simulink model "Quadcopter_nonlinear_Roll_Pitch"  (R2020a)
settings: Solver=ode4  StartTime=0.0  StopTime=10.0  FixedStep=0.02  RelTol=1e-3
InitFcn:
  | load_data;
values from neighbouring files (symbols this model uses):
  A1 = (h_cg * g * m_tot) / (m_tot * h_cg^2 + J_xx)    [QuadConstants.m]    (also in roll_parameter_estimation_result.m = 4.62576573735; roll_pitch_parameter_estimation.m = 6.52172868745)
  A3 = (b * d_cg) / (m_tot * h_cg^2 + J_xx)    [QuadConstants.m]    (also in roll_parameter_estimation_result.m = 5.47149559873e-05; roll_pitch_parameter_estimation.m = 5.18692283683e-05)
  A4 = (J_R) / (m_tot * h_cg^2 + J_xx)    [QuadConstants.m]    (also in roll_pitch_parameter_estimation.m = 0.00249993776858)
  A5 = (m1 * g * miu_k * r_x) / (m_tot * h_cg^2 + J_xx)    [QuadConstants.m]    (also in roll_parameter_estimation_result.m = 0.0125335544194; roll_pitch_parameter_estimation.m = -0.25964581952)
  A6 = 0.628891443554123    (= 0.628891443554)    [roll_parameter_estimation_result.m]    (also in roll_pitch_parameter_estimation.m = 1.37409031322)
  b = 3.12e-5    (= 3.12e-05)    [QuadParameter.m]    (also in QuadParameter_v1.m = 3.13e-05)
  B6 = 3.49728    [pitch_parameter_estiation_result.m]    (also in pitch_parameter_estiation_result_II.m = 4.42876359313; roll_pitch_parameter_estimation.m = 4.42876359313)
  d_cg = 0.295    [QuadParameter.m]    (also in QuadParameter_v1.m = 0.2)
  g = 9.81    [QuadParameter.m]
  h_cg = 0.0078    [QuadParameter.m]
  init_I = data_I(1, :)    [PS_I.m]
  init_II = data_II(1, :)    [PS_II.m]
  init_III = data_III(1, :)    [PS_III.m]
  init_IV = data_IV(1, :)    [PS_IV.m]
  init_IX = data_IX(1, :)    [PS_IX.m]
  init_V = data_V(1, :)    [PS_V.m]
  init_VI = data_VI(1, :)    [PS_VI.m]
  init_VII = data_VII(1, :)    [PS_VII.m]
  init_X = data_X(1, :)    [PS_X.m]
  J_R = 4.439e-5    (= 4.439e-05)    [QuadParameter.m]
  J_yy = 0.03066    [QuadParameter.m]
  m2 = 1.074    [QuadParameter.m]
  m_tot = 1.774    [QuadParameter.m]
  miu_k = 0.002    [QuadParameter.m]
  Omega_I = Omega(1, :)    [PS_I.m]
  Omega_II = Omega(1, :)    [PS_II.m]
  Omega_III = Omega(1, :)    [PS_III.m]
  Omega_IV = Omega(1, :)    [PS_IV.m]
  Omega_IX = Omega(1, :)    [PS_IX.m]
  Omega_V = Omega(1, :)    [PS_V.m]
  Omega_VI = Omega(1, :)    [PS_VI.m]
  Omega_VII = Omega(1, :)    [PS_VII.m]
  Omega_X = Omega(1, :)    [PS_X.m]
  r_y = 0.01    [QuadParameter.m]
undefined symbols (not defined in the file or in its folder): magnitude
(part 2 of 3)

== system Quadcopter_nonlinear_Roll_Pitch/Quadcopter 2DOF (Roll-Pitch) Nonlinear System1/Quad System/dot(x1)/1 ==
  X : Inport
  Demux : Demux  Outputs=3
  Selector : Selector  InputPortWidth=4  IndexOptions=Index vector (dialog)  Indices=[1 2 4]  OutputSizes=1
  Subsystem : Subsystem
  x5sin(x1)tan(x2) : Outport
  wires:
  Demux/2 -> Subsystem/2(x2)  "x2"
  X/1 -> Selector/1  "x"
  Demux/1 -> Subsystem/1(x1)  "x1"
  Demux/3 -> Subsystem/3(x5)  "x5"
  Subsystem/1(x5sin(x1)tan(x2)) -> x5sin(x1)tan(x2)/1
  Selector/1 -> Demux/1

== system Quadcopter_nonlinear_Roll_Pitch/Quadcopter 2DOF (Roll-Pitch) Nonlinear System1/Quad System/dot(x1)/Subsystem1 ==
  X : Inport
  Selector : Selector  InputPortWidth=4  IndexOptions=Index vector (dialog)  Indices=[3]  OutputSizes=1
  x4 : Outport
  wires:
  Selector/1 -> x4/1
  X/1 -> Selector/1

== system Quadcopter_nonlinear_Roll_Pitch/Quadcopter 2DOF (Roll-Pitch) Nonlinear System1/Quad System/dot(x2)/1 ==
  X : Inport
  Demux : Demux  Outputs=2
  Selector : Selector  InputPortWidth=4  IndexOptions=Index vector (dialog)  Indices=[1 4]  OutputSizes=1
  Subsystem : Subsystem
  x5cos(x1) : Outport
  wires:
  X/1 -> Selector/1  "x"
  Demux/1 -> Subsystem/1(x1)  "x1"
  Demux/2 -> Subsystem/2(x5)  "x5"
  Subsystem/1(Out1) -> x5cos(x1)/1
  Selector/1 -> Demux/1

== system Quadcopter_nonlinear_Roll_Pitch/Quadcopter 2DOF (Roll-Pitch) Nonlinear System1/Quad System/dot(x4)/1 ==
  X : Inport
  Demux : Demux  Outputs=2
  Selector : Selector  InputPortWidth=4  IndexOptions=Index vector (dialog)  Indices=[1 2]  OutputSizes=1
  Subsystem : Subsystem
  A1cos(x2)sin(x1) : Outport
  wires:
  Demux/1 -> Subsystem/1(x1)  "x1"
  Subsystem/1(A1cos(x2)sin(x1)) -> A1cos(x2)sin(x1)/1
  Demux/2 -> Subsystem/2(x2)  "x2"
  X/1 -> Selector/1  "x"
  Selector/1 -> Demux/1

== system Quadcopter_nonlinear_Roll_Pitch/Quadcopter 2DOF (Roll-Pitch) Nonlinear System1/Quad System/dot(x4)/2 ==
  X : Inport
  Selector : Selector  InputPortWidth=4  IndexOptions=Index vector (dialog)  Indices=[1]  OutputSizes=1
  Subsystem : Subsystem
  Moment a : Outport
  wires:
  Selector/1 -> Subsystem/1(x1)  "x1"
  Subsystem/1(Moment_a) -> Moment a/1
  X/1 -> Selector/1  "x"

== system Quadcopter_nonlinear_Roll_Pitch/Quadcopter 2DOF (Roll-Pitch) Nonlinear System1/Quad System/dot(x4)/3 ==
  X : Inport
  Selector : Selector  InputPortWidth=4  IndexOptions=Index vector (dialog)  Indices=[3]  OutputSizes=1
  Subsystem : Subsystem
  "-A5x4/|x4| " : Outport
  wires:
  Subsystem/1("-A5x4/|x4| ") -> "-A5x4/|x4| "/1
  Selector/1 -> Subsystem/1(x4)
  X/1 -> Selector/1  "x"

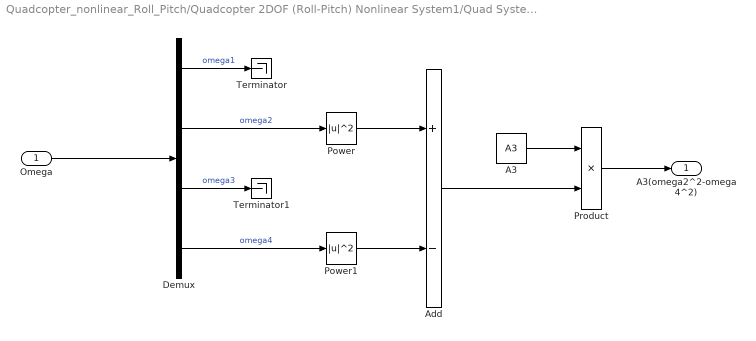
== system Quadcopter_nonlinear_Roll_Pitch/Quadcopter 2DOF (Roll-Pitch) Nonlinear System1/Quad System/dot(x4)/Subsystem ==
  Omega : Inport
  A3 : Constant  Value=A3
  Add : Sum  Inputs=+-
  Demux : Demux
  Power : Math  Operator=magnitude^2  SaturateOnIntegerOverflow=on
  Power1 : Math  Operator=magnitude^2  SaturateOnIntegerOverflow=on
  Product : Product
  Terminator : Terminator
  Terminator1 : Terminator
  A3(omega2^2-omega4^2) : Outport
  wires:
  Product/1 -> A3(omega2^2-omega4^2)/1
  Power1/1 -> Add/2
  Demux/2 -> Power/1  "omega2"
  Demux/4 -> Power1/1  "omega4"
  Add/1 -> Product/2
  Power/1 -> Add/1
  A3/1 -> Product/1
  Omega/1 -> Demux/1
  Demux/3 -> Terminator1/1  "omega3"
  Demux/1 -> Terminator/1  "omega1"

== system Quadcopter_nonlinear_Roll_Pitch/Quadcopter 2DOF (Roll-Pitch) Nonlinear System1/Quad System/dot(x4)/Subsystem1 ==
  X : Inport
  Omega : Inport  Port=2
  A4 : Constant  Value=A4
  Add : Sum  Inputs=+-+-
  Demux : Demux
  Product : Product  Inputs=3
  Selector : Selector  InputPortWidth=4  IndexOptions=Index vector (dialog)  Indices=[4]  OutputSizes=1
  A4x5(omega1-omega2+omega3-omega4) : Outport
  wires:
  Omega/1 -> Demux/1
  Demux/1 -> Add/1  "omega1"
  Demux/2 -> Add/2  "omega2"
  Demux/3 -> Add/3  "omega3"
  Demux/4 -> Add/4  "omega4"
  Add/1 -> Product/1
  A4/1 -> Product/2
  Product/1 -> A4x5(omega1-omega2+omega3-omega4)/1
  Selector/1 -> Product/3
  X/1 -> Selector/1  "x"

== system Quadcopter_nonlinear_Roll_Pitch/Quadcopter 2DOF (Roll-Pitch) Nonlinear System1/Quad System/dot(x5)/1 ==
  X : Inport
  Selector : Selector  InputPortWidth=4  IndexOptions=Index vector (dialog)  Indices=[2]  OutputSizes=1
  Subsystem : Subsystem
  B1sin(x2) : Outport
  wires:
  Subsystem/1(B1sin(x2)) -> B1sin(x2)/1
  Selector/1 -> Subsystem/1(x2)
  X/1 -> Selector/1  "x"

== system Quadcopter_nonlinear_Roll_Pitch/Quadcopter 2DOF (Roll-Pitch) Nonlinear System1/Quad System/dot(x5)/2 ==
  X : Inport
  Selector : Selector  InputPortWidth=4  IndexOptions=Index vector (dialog)  Indices=[2]  OutputSizes=1
  Subsystem : Subsystem
  Moment_a : Outport
  wires:
  X/1 -> Selector/1  "x"
  Subsystem/1(moment_a) -> Moment_a/1
  Selector/1 -> Subsystem/1(In1)

== system Quadcopter_nonlinear_Roll_Pitch/Quadcopter 2DOF (Roll-Pitch) Nonlinear System1/Quad System/dot(x5)/3 ==
  X : Inport
  Selector : Selector  InputPortWidth=4  IndexOptions=Index vector (dialog)  Indices=[4]  OutputSizes=1
  Subsystem : Subsystem
  "-B5x5/|x5| " : Outport
  wires:
  Selector/1 -> Subsystem/1(x5)  "x5"
  Subsystem/1("-B5x5/|x5| ") -> "-B5x5/|x5| "/1
  X/1 -> Selector/1  "x"

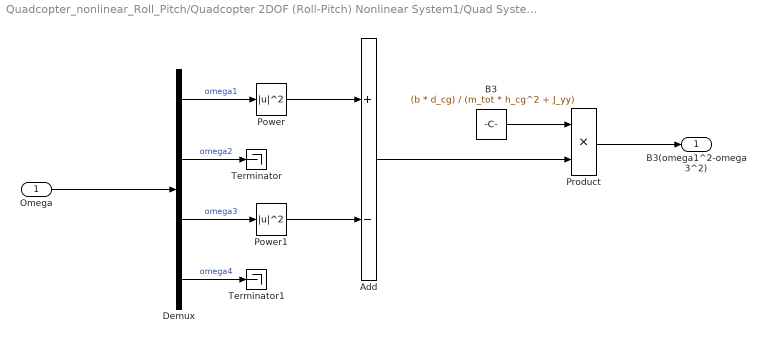
== system Quadcopter_nonlinear_Roll_Pitch/Quadcopter 2DOF (Roll-Pitch) Nonlinear System1/Quad System/dot(x5)/Subsystem ==
  Omega : Inport
  Add : Sum  Inputs=+-
  B3 : Constant  Value=(b * d_cg) / (m_tot * h_cg^2 + J_yy)
  Demux : Demux
  Power : Math  Operator=magnitude^2  SaturateOnIntegerOverflow=on
  Power1 : Math  Operator=magnitude^2  SaturateOnIntegerOverflow=on
  Product : Product
  Terminator : Terminator
  Terminator1 : Terminator
  B3(omega1^2-omega3^2) : Outport
  wires:
  Product/1 -> B3(omega1^2-omega3^2)/1
  Power1/1 -> Add/2
  Add/1 -> Product/2
  Power/1 -> Add/1
  B3/1 -> Product/1
  Omega/1 -> Demux/1
  Demux/3 -> Power1/1  "omega3"
  Demux/1 -> Power/1  "omega1"
  Demux/2 -> Terminator/1  "omega2"
  Demux/4 -> Terminator1/1  "omega4"

== system Quadcopter_nonlinear_Roll_Pitch/Quadcopter 2DOF (Roll-Pitch) Nonlinear System1/Quad System/dot(x5)/Subsystem1 ==
  X : Inport
  Omega : Inport  Port=2
  Add : Sum  Inputs=+-+-
  B4 : Constant  Value=(-J_R) / (m_tot * h_cg^2 + J_yy)
  Demux : Demux
  Product : Product  Inputs=3
  Selector : Selector  InputPortWidth=4  IndexOptions=Index vector (dialog)  Indices=[3]  OutputSizes=1
  B4x4(omega1-omega2+omega3-omega4) : Outport
  wires:
  Omega/1 -> Demux/1
  Demux/1 -> Add/1  "omega1"
  Demux/2 -> Add/2  "omega2"
  Demux/3 -> Add/3  "omega3"
  Demux/4 -> Add/4  "omega4"
  Add/1 -> Product/1
  B4/1 -> Product/2
  Product/1 -> B4x4(omega1-omega2+omega3-omega4)/1
  Selector/1 -> Product/3
  X/1 -> Selector/1  "x"

== system Quadcopter_nonlinear_Roll_Pitch/Quadcopter 2DOF (Roll-Pitch) Nonlinear System2/Quad System/dot(x1)/1 ==
  X : Inport
  Demux : Demux  Outputs=3
  Selector : Selector  InputPortWidth=4  IndexOptions=Index vector (dialog)  Indices=[1 2 4]  OutputSizes=1
  Subsystem : Subsystem
  x5sin(x1)tan(x2) : Outport
  wires:
  Demux/2 -> Subsystem/2(x2)  "x2"
  X/1 -> Selector/1  "x"
  Demux/1 -> Subsystem/1(x1)  "x1"
  Demux/3 -> Subsystem/3(x5)  "x5"
  Subsystem/1(x5sin(x1)tan(x2)) -> x5sin(x1)tan(x2)/1
  Selector/1 -> Demux/1

== system Quadcopter_nonlinear_Roll_Pitch/Quadcopter 2DOF (Roll-Pitch) Nonlinear System2/Quad System/dot(x1)/Subsystem1 ==
  X : Inport
  Selector : Selector  InputPortWidth=4  IndexOptions=Index vector (dialog)  Indices=[3]  OutputSizes=1
  x4 : Outport
  wires:
  Selector/1 -> x4/1
  X/1 -> Selector/1

== system Quadcopter_nonlinear_Roll_Pitch/Quadcopter 2DOF (Roll-Pitch) Nonlinear System2/Quad System/dot(x2)/1 ==
  X : Inport
  Demux : Demux  Outputs=2
  Selector : Selector  InputPortWidth=4  IndexOptions=Index vector (dialog)  Indices=[1 4]  OutputSizes=1
  Subsystem : Subsystem
  x5cos(x1) : Outport
  wires:
  X/1 -> Selector/1  "x"
  Demux/1 -> Subsystem/1(x1)  "x1"
  Demux/2 -> Subsystem/2(x5)  "x5"
  Subsystem/1(Out1) -> x5cos(x1)/1
  Selector/1 -> Demux/1

== system Quadcopter_nonlinear_Roll_Pitch/Quadcopter 2DOF (Roll-Pitch) Nonlinear System2/Quad System/dot(x4)/1 ==
  X : Inport
  Demux : Demux  Outputs=2
  Selector : Selector  InputPortWidth=4  IndexOptions=Index vector (dialog)  Indices=[1 2]  OutputSizes=1
  Subsystem : Subsystem
  A1cos(x2)sin(x1) : Outport
  wires:
  Demux/1 -> Subsystem/1(x1)  "x1"
  Subsystem/1(A1cos(x2)sin(x1)) -> A1cos(x2)sin(x1)/1
  Demux/2 -> Subsystem/2(x2)  "x2"
  X/1 -> Selector/1  "x"
  Selector/1 -> Demux/1

== system Quadcopter_nonlinear_Roll_Pitch/Quadcopter 2DOF (Roll-Pitch) Nonlinear System2/Quad System/dot(x4)/2 ==
  X : Inport
  Selector : Selector  InputPortWidth=4  IndexOptions=Index vector (dialog)  Indices=[1]  OutputSizes=1
  Subsystem : Subsystem
  Moment a : Outport
  wires:
  Selector/1 -> Subsystem/1(x1)  "x1"
  Subsystem/1(Moment_a) -> Moment a/1
  X/1 -> Selector/1  "x"

== system Quadcopter_nonlinear_Roll_Pitch/Quadcopter 2DOF (Roll-Pitch) Nonlinear System2/Quad System/dot(x4)/3 ==
  X : Inport
  Selector : Selector  InputPortWidth=4  IndexOptions=Index vector (dialog)  Indices=[3]  OutputSizes=1
  Subsystem : Subsystem
  "-A5x4/|x4| " : Outport
  wires:
  Subsystem/1("-A5x4/|x4| ") -> "-A5x4/|x4| "/1
  Selector/1 -> Subsystem/1(x4)
  X/1 -> Selector/1  "x"

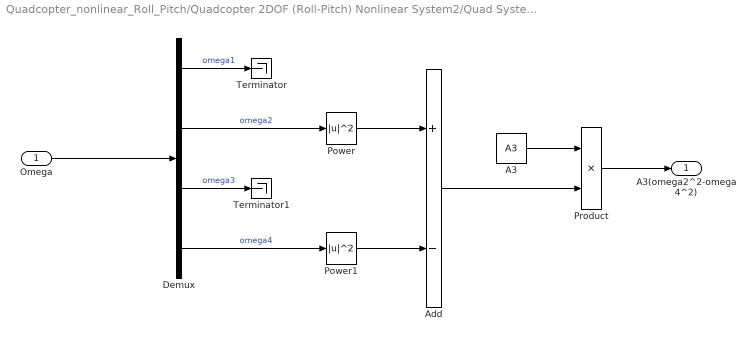
== system Quadcopter_nonlinear_Roll_Pitch/Quadcopter 2DOF (Roll-Pitch) Nonlinear System2/Quad System/dot(x4)/Subsystem ==
  Omega : Inport
  A3 : Constant  Value=A3
  Add : Sum  Inputs=+-
  Demux : Demux
  Power : Math  Operator=magnitude^2  SaturateOnIntegerOverflow=on
  Power1 : Math  Operator=magnitude^2  SaturateOnIntegerOverflow=on
  Product : Product
  Terminator : Terminator
  Terminator1 : Terminator
  A3(omega2^2-omega4^2) : Outport
  wires:
  Product/1 -> A3(omega2^2-omega4^2)/1
  Power1/1 -> Add/2
  Demux/2 -> Power/1  "omega2"
  Demux/4 -> Power1/1  "omega4"
  Add/1 -> Product/2
  Power/1 -> Add/1
  A3/1 -> Product/1
  Omega/1 -> Demux/1
  Demux/3 -> Terminator1/1  "omega3"
  Demux/1 -> Terminator/1  "omega1"

== system Quadcopter_nonlinear_Roll_Pitch/Quadcopter 2DOF (Roll-Pitch) Nonlinear System2/Quad System/dot(x4)/Subsystem1 ==
  X : Inport
  Omega : Inport  Port=2
  A4 : Constant  Value=A4
  Add : Sum  Inputs=+-+-
  Demux : Demux
  Product : Product  Inputs=3
  Selector : Selector  InputPortWidth=4  IndexOptions=Index vector (dialog)  Indices=[4]  OutputSizes=1
  A4x5(omega1-omega2+omega3-omega4) : Outport
  wires:
  Omega/1 -> Demux/1
  Demux/1 -> Add/1  "omega1"
  Demux/2 -> Add/2  "omega2"
  Demux/3 -> Add/3  "omega3"
  Demux/4 -> Add/4  "omega4"
  Add/1 -> Product/1
  A4/1 -> Product/2
  Product/1 -> A4x5(omega1-omega2+omega3-omega4)/1
  Selector/1 -> Product/3
  X/1 -> Selector/1  "x"

== system Quadcopter_nonlinear_Roll_Pitch/Quadcopter 2DOF (Roll-Pitch) Nonlinear System2/Quad System/dot(x5)/1 ==
  X : Inport
  Selector : Selector  InputPortWidth=4  IndexOptions=Index vector (dialog)  Indices=[2]  OutputSizes=1
  Subsystem : Subsystem
  B1sin(x2) : Outport
  wires:
  Subsystem/1(B1sin(x2)) -> B1sin(x2)/1
  Selector/1 -> Subsystem/1(x2)
  X/1 -> Selector/1  "x"

== system Quadcopter_nonlinear_Roll_Pitch/Quadcopter 2DOF (Roll-Pitch) Nonlinear System2/Quad System/dot(x5)/2 ==
  X : Inport
  Selector : Selector  InputPortWidth=4  IndexOptions=Index vector (dialog)  Indices=[2]  OutputSizes=1
  Subsystem : Subsystem
  Moment_a : Outport
  wires:
  X/1 -> Selector/1  "x"
  Subsystem/1(moment_a) -> Moment_a/1
  Selector/1 -> Subsystem/1(In1)

== system Quadcopter_nonlinear_Roll_Pitch/Quadcopter 2DOF (Roll-Pitch) Nonlinear System2/Quad System/dot(x5)/3 ==
  X : Inport
  Selector : Selector  InputPortWidth=4  IndexOptions=Index vector (dialog)  Indices=[4]  OutputSizes=1
  Subsystem : Subsystem
  "-B5x5/|x5| " : Outport
  wires:
  Selector/1 -> Subsystem/1(x5)  "x5"
  Subsystem/1("-B5x5/|x5| ") -> "-B5x5/|x5| "/1
  X/1 -> Selector/1  "x"

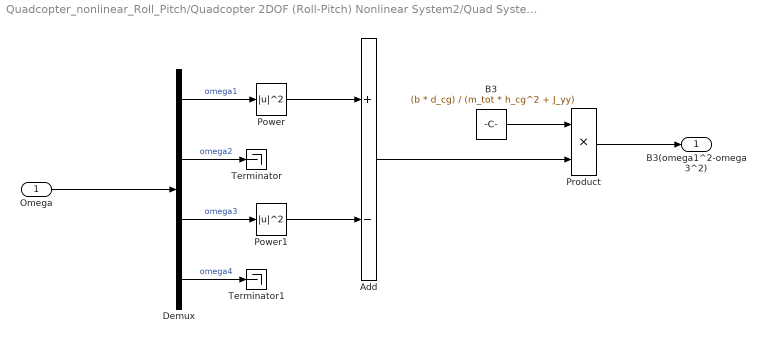
== system Quadcopter_nonlinear_Roll_Pitch/Quadcopter 2DOF (Roll-Pitch) Nonlinear System2/Quad System/dot(x5)/Subsystem ==
  Omega : Inport
  Add : Sum  Inputs=+-
  B3 : Constant  Value=(b * d_cg) / (m_tot * h_cg^2 + J_yy)
  Demux : Demux
  Power : Math  Operator=magnitude^2  SaturateOnIntegerOverflow=on
  Power1 : Math  Operator=magnitude^2  SaturateOnIntegerOverflow=on
  Product : Product
  Terminator : Terminator
  Terminator1 : Terminator
  B3(omega1^2-omega3^2) : Outport
  wires:
  Product/1 -> B3(omega1^2-omega3^2)/1
  Power1/1 -> Add/2
  Add/1 -> Product/2
  Power/1 -> Add/1
  B3/1 -> Product/1
  Omega/1 -> Demux/1
  Demux/3 -> Power1/1  "omega3"
  Demux/1 -> Power/1  "omega1"
  Demux/2 -> Terminator/1  "omega2"
  Demux/4 -> Terminator1/1  "omega4"

== system Quadcopter_nonlinear_Roll_Pitch/Quadcopter 2DOF (Roll-Pitch) Nonlinear System2/Quad System/dot(x5)/Subsystem1 ==
  X : Inport
  Omega : Inport  Port=2
  Add : Sum  Inputs=+-+-
  B4 : Constant  Value=(-J_R) / (m_tot * h_cg^2 + J_yy)
  Demux : Demux
  Product : Product  Inputs=3
  Selector : Selector  InputPortWidth=4  IndexOptions=Index vector (dialog)  Indices=[3]  OutputSizes=1
  B4x4(omega1-omega2+omega3-omega4) : Outport
  wires:
  Omega/1 -> Demux/1
  Demux/1 -> Add/1  "omega1"
  Demux/2 -> Add/2  "omega2"
  Demux/3 -> Add/3  "omega3"
  Demux/4 -> Add/4  "omega4"
  Add/1 -> Product/1
  B4/1 -> Product/2
  Product/1 -> B4x4(omega1-omega2+omega3-omega4)/1
  Selector/1 -> Product/3
  X/1 -> Selector/1  "x"

== system Quadcopter_nonlinear_Roll_Pitch/Quadcopter 2DOF (Roll-Pitch) Nonlinear System3/Quad System/dot(x1)/1 ==
  X : Inport
  Demux : Demux  Outputs=3
  Selector : Selector  InputPortWidth=4  IndexOptions=Index vector (dialog)  Indices=[1 2 4]  OutputSizes=1
  Subsystem : Subsystem
  x5sin(x1)tan(x2) : Outport
  wires:
  Demux/2 -> Subsystem/2(x2)  "x2"
  X/1 -> Selector/1  "x"
  Demux/1 -> Subsystem/1(x1)  "x1"
  Demux/3 -> Subsystem/3(x5)  "x5"
  Subsystem/1(x5sin(x1)tan(x2)) -> x5sin(x1)tan(x2)/1
  Selector/1 -> Demux/1

== system Quadcopter_nonlinear_Roll_Pitch/Quadcopter 2DOF (Roll-Pitch) Nonlinear System3/Quad System/dot(x1)/Subsystem1 ==
  X : Inport
  Selector : Selector  InputPortWidth=4  IndexOptions=Index vector (dialog)  Indices=[3]  OutputSizes=1
  x4 : Outport
  wires:
  Selector/1 -> x4/1
  X/1 -> Selector/1

== system Quadcopter_nonlinear_Roll_Pitch/Quadcopter 2DOF (Roll-Pitch) Nonlinear System3/Quad System/dot(x2)/1 ==
  X : Inport
  Demux : Demux  Outputs=2
  Selector : Selector  InputPortWidth=4  IndexOptions=Index vector (dialog)  Indices=[1 4]  OutputSizes=1
  Subsystem : Subsystem
  x5cos(x1) : Outport
  wires:
  X/1 -> Selector/1  "x"
  Demux/1 -> Subsystem/1(x1)  "x1"
  Demux/2 -> Subsystem/2(x5)  "x5"
  Subsystem/1(Out1) -> x5cos(x1)/1
  Selector/1 -> Demux/1

== system Quadcopter_nonlinear_Roll_Pitch/Quadcopter 2DOF (Roll-Pitch) Nonlinear System3/Quad System/dot(x4)/1 ==
  X : Inport
  Demux : Demux  Outputs=2
  Selector : Selector  InputPortWidth=4  IndexOptions=Index vector (dialog)  Indices=[1 2]  OutputSizes=1
  Subsystem : Subsystem
  A1cos(x2)sin(x1) : Outport
  wires:
  Demux/1 -> Subsystem/1(x1)  "x1"
  Subsystem/1(A1cos(x2)sin(x1)) -> A1cos(x2)sin(x1)/1
  Demux/2 -> Subsystem/2(x2)  "x2"
  X/1 -> Selector/1  "x"
  Selector/1 -> Demux/1

== system Quadcopter_nonlinear_Roll_Pitch/Quadcopter 2DOF (Roll-Pitch) Nonlinear System3/Quad System/dot(x4)/2 ==
  X : Inport
  Selector : Selector  InputPortWidth=4  IndexOptions=Index vector (dialog)  Indices=[1]  OutputSizes=1
  Subsystem : Subsystem
  Moment a : Outport
  wires:
  Selector/1 -> Subsystem/1(x1)  "x1"
  Subsystem/1(Moment_a) -> Moment a/1
  X/1 -> Selector/1  "x"

== system Quadcopter_nonlinear_Roll_Pitch/Quadcopter 2DOF (Roll-Pitch) Nonlinear System3/Quad System/dot(x4)/3 ==
  X : Inport
  Selector : Selector  InputPortWidth=4  IndexOptions=Index vector (dialog)  Indices=[3]  OutputSizes=1
  Subsystem : Subsystem
  "-A5x4/|x4| " : Outport
  wires:
  Subsystem/1("-A5x4/|x4| ") -> "-A5x4/|x4| "/1
  Selector/1 -> Subsystem/1(x4)
  X/1 -> Selector/1  "x"

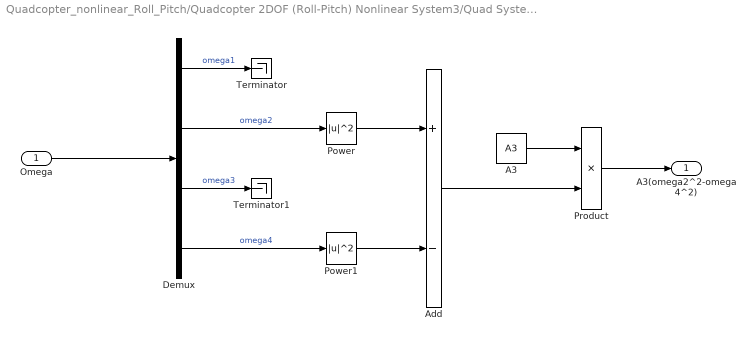
== system Quadcopter_nonlinear_Roll_Pitch/Quadcopter 2DOF (Roll-Pitch) Nonlinear System3/Quad System/dot(x4)/Subsystem ==
  Omega : Inport
  A3 : Constant  Value=A3
  Add : Sum  Inputs=+-
  Demux : Demux
  Power : Math  Operator=magnitude^2  SaturateOnIntegerOverflow=on
  Power1 : Math  Operator=magnitude^2  SaturateOnIntegerOverflow=on
  Product : Product
  Terminator : Terminator
  Terminator1 : Terminator
  A3(omega2^2-omega4^2) : Outport
  wires:
  Product/1 -> A3(omega2^2-omega4^2)/1
  Power1/1 -> Add/2
  Demux/2 -> Power/1  "omega2"
  Demux/4 -> Power1/1  "omega4"
  Add/1 -> Product/2
  Power/1 -> Add/1
  A3/1 -> Product/1
  Omega/1 -> Demux/1
  Demux/3 -> Terminator1/1  "omega3"
  Demux/1 -> Terminator/1  "omega1"

== system Quadcopter_nonlinear_Roll_Pitch/Quadcopter 2DOF (Roll-Pitch) Nonlinear System3/Quad System/dot(x4)/Subsystem1 ==
  X : Inport
  Omega : Inport  Port=2
  A4 : Constant  Value=A4
  Add : Sum  Inputs=+-+-
  Demux : Demux
  Product : Product  Inputs=3
  Selector : Selector  InputPortWidth=4  IndexOptions=Index vector (dialog)  Indices=[4]  OutputSizes=1
  A4x5(omega1-omega2+omega3-omega4) : Outport
  wires:
  Omega/1 -> Demux/1
  Demux/1 -> Add/1  "omega1"
  Demux/2 -> Add/2  "omega2"
  Demux/3 -> Add/3  "omega3"
  Demux/4 -> Add/4  "omega4"
  Add/1 -> Product/1
  A4/1 -> Product/2
  Product/1 -> A4x5(omega1-omega2+omega3-omega4)/1
  Selector/1 -> Product/3
  X/1 -> Selector/1  "x"

== system Quadcopter_nonlinear_Roll_Pitch/Quadcopter 2DOF (Roll-Pitch) Nonlinear System3/Quad System/dot(x5)/1 ==
  X : Inport
  Selector : Selector  InputPortWidth=4  IndexOptions=Index vector (dialog)  Indices=[2]  OutputSizes=1
  Subsystem : Subsystem
  B1sin(x2) : Outport
  wires:
  Subsystem/1(B1sin(x2)) -> B1sin(x2)/1
  Selector/1 -> Subsystem/1(x2)
  X/1 -> Selector/1  "x"

== system Quadcopter_nonlinear_Roll_Pitch/Quadcopter 2DOF (Roll-Pitch) Nonlinear System3/Quad System/dot(x5)/2 ==
  X : Inport
  Selector : Selector  InputPortWidth=4  IndexOptions=Index vector (dialog)  Indices=[2]  OutputSizes=1
  Subsystem : Subsystem
  Moment_a : Outport
  wires:
  X/1 -> Selector/1  "x"
  Subsystem/1(moment_a) -> Moment_a/1
  Selector/1 -> Subsystem/1(In1)

== system Quadcopter_nonlinear_Roll_Pitch/Quadcopter 2DOF (Roll-Pitch) Nonlinear System3/Quad System/dot(x5)/3 ==
  X : Inport
  Selector : Selector  InputPortWidth=4  IndexOptions=Index vector (dialog)  Indices=[4]  OutputSizes=1
  Subsystem : Subsystem
  "-B5x5/|x5| " : Outport
  wires:
  Selector/1 -> Subsystem/1(x5)  "x5"
  Subsystem/1("-B5x5/|x5| ") -> "-B5x5/|x5| "/1
  X/1 -> Selector/1  "x"

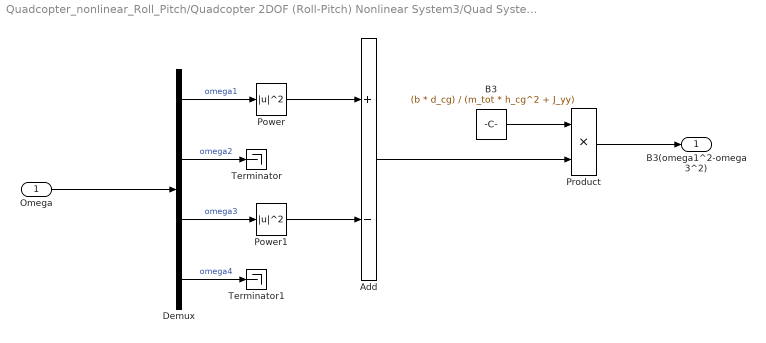
== system Quadcopter_nonlinear_Roll_Pitch/Quadcopter 2DOF (Roll-Pitch) Nonlinear System3/Quad System/dot(x5)/Subsystem ==
  Omega : Inport
  Add : Sum  Inputs=+-
  B3 : Constant  Value=(b * d_cg) / (m_tot * h_cg^2 + J_yy)
  Demux : Demux
  Power : Math  Operator=magnitude^2  SaturateOnIntegerOverflow=on
  Power1 : Math  Operator=magnitude^2  SaturateOnIntegerOverflow=on
  Product : Product
  Terminator : Terminator
  Terminator1 : Terminator
  B3(omega1^2-omega3^2) : Outport
  wires:
  Product/1 -> B3(omega1^2-omega3^2)/1
  Power1/1 -> Add/2
  Add/1 -> Product/2
  Power/1 -> Add/1
  B3/1 -> Product/1
  Omega/1 -> Demux/1
  Demux/3 -> Power1/1  "omega3"
  Demux/1 -> Power/1  "omega1"
  Demux/2 -> Terminator/1  "omega2"
  Demux/4 -> Terminator1/1  "omega4"

== system Quadcopter_nonlinear_Roll_Pitch/Quadcopter 2DOF (Roll-Pitch) Nonlinear System3/Quad System/dot(x5)/Subsystem1 ==
  X : Inport
  Omega : Inport  Port=2
  Add : Sum  Inputs=+-+-
  B4 : Constant  Value=(-J_R) / (m_tot * h_cg^2 + J_yy)
  Demux : Demux
  Product : Product  Inputs=3
  Selector : Selector  InputPortWidth=4  IndexOptions=Index vector (dialog)  Indices=[3]  OutputSizes=1
  B4x4(omega1-omega2+omega3-omega4) : Outport
  wires:
  Omega/1 -> Demux/1
  Demux/1 -> Add/1  "omega1"
  Demux/2 -> Add/2  "omega2"
  Demux/3 -> Add/3  "omega3"
  Demux/4 -> Add/4  "omega4"
  Add/1 -> Product/1
  B4/1 -> Product/2
  Product/1 -> B4x4(omega1-omega2+omega3-omega4)/1
  Selector/1 -> Product/3
  X/1 -> Selector/1  "x"

== system Quadcopter_nonlinear_Roll_Pitch/Quadcopter 2DOF (Roll-Pitch) Nonlinear System4/Quad System/dot(x1)/1 ==
  X : Inport
  Demux : Demux  Outputs=3
  Selector : Selector  InputPortWidth=4  IndexOptions=Index vector (dialog)  Indices=[1 2 4]  OutputSizes=1
  Subsystem : Subsystem
  x5sin(x1)tan(x2) : Outport
  wires:
  Demux/2 -> Subsystem/2(x2)  "x2"
  X/1 -> Selector/1  "x"
  Demux/1 -> Subsystem/1(x1)  "x1"
  Demux/3 -> Subsystem/3(x5)  "x5"
  Subsystem/1(x5sin(x1)tan(x2)) -> x5sin(x1)tan(x2)/1
  Selector/1 -> Demux/1

== system Quadcopter_nonlinear_Roll_Pitch/Quadcopter 2DOF (Roll-Pitch) Nonlinear System4/Quad System/dot(x1)/Subsystem1 ==
  X : Inport
  Selector : Selector  InputPortWidth=4  IndexOptions=Index vector (dialog)  Indices=[3]  OutputSizes=1
  x4 : Outport
  wires:
  Selector/1 -> x4/1
  X/1 -> Selector/1

== system Quadcopter_nonlinear_Roll_Pitch/Quadcopter 2DOF (Roll-Pitch) Nonlinear System4/Quad System/dot(x2)/1 ==
  X : Inport
  Demux : Demux  Outputs=2
  Selector : Selector  InputPortWidth=4  IndexOptions=Index vector (dialog)  Indices=[1 4]  OutputSizes=1
  Subsystem : Subsystem
  x5cos(x1) : Outport
  wires:
  X/1 -> Selector/1  "x"
  Demux/1 -> Subsystem/1(x1)  "x1"
  Demux/2 -> Subsystem/2(x5)  "x5"
  Subsystem/1(Out1) -> x5cos(x1)/1
  Selector/1 -> Demux/1

== system Quadcopter_nonlinear_Roll_Pitch/Quadcopter 2DOF (Roll-Pitch) Nonlinear System4/Quad System/dot(x4)/1 ==
  X : Inport
  Demux : Demux  Outputs=2
  Selector : Selector  InputPortWidth=4  IndexOptions=Index vector (dialog)  Indices=[1 2]  OutputSizes=1
  Subsystem : Subsystem
  A1cos(x2)sin(x1) : Outport
  wires:
  Demux/1 -> Subsystem/1(x1)  "x1"
  Subsystem/1(A1cos(x2)sin(x1)) -> A1cos(x2)sin(x1)/1
  Demux/2 -> Subsystem/2(x2)  "x2"
  X/1 -> Selector/1  "x"
  Selector/1 -> Demux/1

== system Quadcopter_nonlinear_Roll_Pitch/Quadcopter 2DOF (Roll-Pitch) Nonlinear System4/Quad System/dot(x4)/2 ==
  X : Inport
  Selector : Selector  InputPortWidth=4  IndexOptions=Index vector (dialog)  Indices=[1]  OutputSizes=1
  Subsystem : Subsystem
  Moment a : Outport
  wires:
  Selector/1 -> Subsystem/1(x1)  "x1"
  Subsystem/1(Moment_a) -> Moment a/1
  X/1 -> Selector/1  "x"

== system Quadcopter_nonlinear_Roll_Pitch/Quadcopter 2DOF (Roll-Pitch) Nonlinear System4/Quad System/dot(x4)/3 ==
  X : Inport
  Selector : Selector  InputPortWidth=4  IndexOptions=Index vector (dialog)  Indices=[3]  OutputSizes=1
  Subsystem : Subsystem
  "-A5x4/|x4| " : Outport
  wires:
  Subsystem/1("-A5x4/|x4| ") -> "-A5x4/|x4| "/1
  Selector/1 -> Subsystem/1(x4)
  X/1 -> Selector/1  "x"

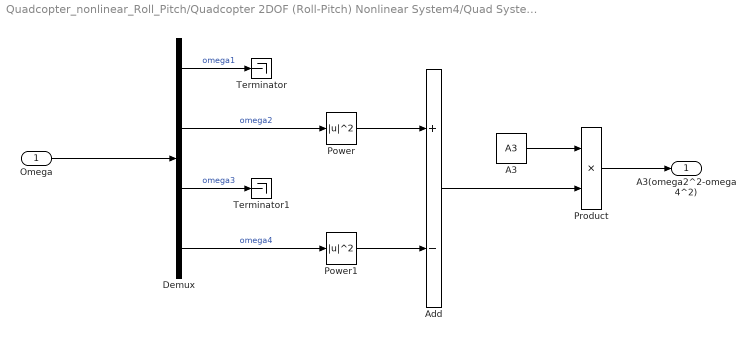
== system Quadcopter_nonlinear_Roll_Pitch/Quadcopter 2DOF (Roll-Pitch) Nonlinear System4/Quad System/dot(x4)/Subsystem ==
  Omega : Inport
  A3 : Constant  Value=A3
  Add : Sum  Inputs=+-
  Demux : Demux
  Power : Math  Operator=magnitude^2  SaturateOnIntegerOverflow=on
  Power1 : Math  Operator=magnitude^2  SaturateOnIntegerOverflow=on
  Product : Product
  Terminator : Terminator
  Terminator1 : Terminator
  A3(omega2^2-omega4^2) : Outport
  wires:
  Product/1 -> A3(omega2^2-omega4^2)/1
  Power1/1 -> Add/2
  Demux/2 -> Power/1  "omega2"
  Demux/4 -> Power1/1  "omega4"
  Add/1 -> Product/2
  Power/1 -> Add/1
  A3/1 -> Product/1
  Omega/1 -> Demux/1
  Demux/3 -> Terminator1/1  "omega3"
  Demux/1 -> Terminator/1  "omega1"

== system Quadcopter_nonlinear_Roll_Pitch/Quadcopter 2DOF (Roll-Pitch) Nonlinear System4/Quad System/dot(x4)/Subsystem1 ==
  X : Inport
  Omega : Inport  Port=2
  A4 : Constant  Value=A4
  Add : Sum  Inputs=+-+-
  Demux : Demux
  Product : Product  Inputs=3
  Selector : Selector  InputPortWidth=4  IndexOptions=Index vector (dialog)  Indices=[4]  OutputSizes=1
  A4x5(omega1-omega2+omega3-omega4) : Outport
  wires:
  Omega/1 -> Demux/1
  Demux/1 -> Add/1  "omega1"
  Demux/2 -> Add/2  "omega2"
  Demux/3 -> Add/3  "omega3"
  Demux/4 -> Add/4  "omega4"
  Add/1 -> Product/1
  A4/1 -> Product/2
  Product/1 -> A4x5(omega1-omega2+omega3-omega4)/1
  Selector/1 -> Product/3
  X/1 -> Selector/1  "x"

== system Quadcopter_nonlinear_Roll_Pitch/Quadcopter 2DOF (Roll-Pitch) Nonlinear System4/Quad System/dot(x5)/1 ==
  X : Inport
  Selector : Selector  InputPortWidth=4  IndexOptions=Index vector (dialog)  Indices=[2]  OutputSizes=1
  Subsystem : Subsystem
  B1sin(x2) : Outport
  wires:
  Subsystem/1(B1sin(x2)) -> B1sin(x2)/1
  Selector/1 -> Subsystem/1(x2)
  X/1 -> Selector/1  "x"

== system Quadcopter_nonlinear_Roll_Pitch/Quadcopter 2DOF (Roll-Pitch) Nonlinear System4/Quad System/dot(x5)/2 ==
  X : Inport
  Selector : Selector  InputPortWidth=4  IndexOptions=Index vector (dialog)  Indices=[2]  OutputSizes=1
  Subsystem : Subsystem
  Moment_a : Outport
  wires:
  X/1 -> Selector/1  "x"
  Subsystem/1(moment_a) -> Moment_a/1
  Selector/1 -> Subsystem/1(In1)

== system Quadcopter_nonlinear_Roll_Pitch/Quadcopter 2DOF (Roll-Pitch) Nonlinear System4/Quad System/dot(x5)/3 ==
  X : Inport
  Selector : Selector  InputPortWidth=4  IndexOptions=Index vector (dialog)  Indices=[4]  OutputSizes=1
  Subsystem : Subsystem
  "-B5x5/|x5| " : Outport
  wires:
  Selector/1 -> Subsystem/1(x5)  "x5"
  Subsystem/1("-B5x5/|x5| ") -> "-B5x5/|x5| "/1
  X/1 -> Selector/1  "x"

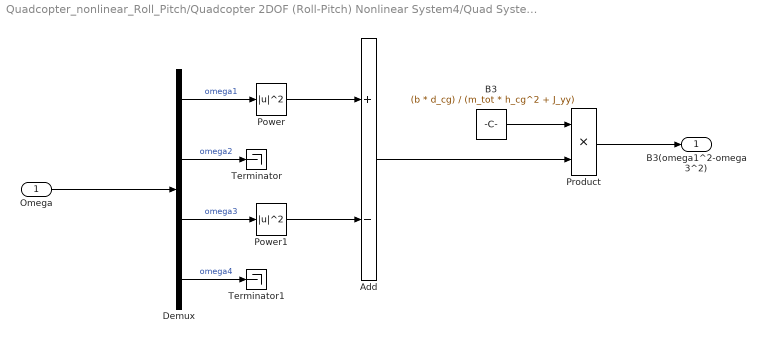
== system Quadcopter_nonlinear_Roll_Pitch/Quadcopter 2DOF (Roll-Pitch) Nonlinear System4/Quad System/dot(x5)/Subsystem ==
  Omega : Inport
  Add : Sum  Inputs=+-
  B3 : Constant  Value=(b * d_cg) / (m_tot * h_cg^2 + J_yy)
  Demux : Demux
  Power : Math  Operator=magnitude^2  SaturateOnIntegerOverflow=on
  Power1 : Math  Operator=magnitude^2  SaturateOnIntegerOverflow=on
  Product : Product
  Terminator : Terminator
  Terminator1 : Terminator
  B3(omega1^2-omega3^2) : Outport
  wires:
  Product/1 -> B3(omega1^2-omega3^2)/1
  Power1/1 -> Add/2
  Add/1 -> Product/2
  Power/1 -> Add/1
  B3/1 -> Product/1
  Omega/1 -> Demux/1
  Demux/3 -> Power1/1  "omega3"
  Demux/1 -> Power/1  "omega1"
  Demux/2 -> Terminator/1  "omega2"
  Demux/4 -> Terminator1/1  "omega4"

== system Quadcopter_nonlinear_Roll_Pitch/Quadcopter 2DOF (Roll-Pitch) Nonlinear System4/Quad System/dot(x5)/Subsystem1 ==
  X : Inport
  Omega : Inport  Port=2
  Add : Sum  Inputs=+-+-
  B4 : Constant  Value=(-J_R) / (m_tot * h_cg^2 + J_yy)
  Demux : Demux
  Product : Product  Inputs=3
  Selector : Selector  InputPortWidth=4  IndexOptions=Index vector (dialog)  Indices=[3]  OutputSizes=1
  B4x4(omega1-omega2+omega3-omega4) : Outport
  wires:
  Omega/1 -> Demux/1
  Demux/1 -> Add/1  "omega1"
  Demux/2 -> Add/2  "omega2"
  Demux/3 -> Add/3  "omega3"
  Demux/4 -> Add/4  "omega4"
  Add/1 -> Product/1
  B4/1 -> Product/2
  Product/1 -> B4x4(omega1-omega2+omega3-omega4)/1
  Selector/1 -> Product/3
  X/1 -> Selector/1  "x"

== system Quadcopter_nonlinear_Roll_Pitch/Quadcopter 2DOF (Roll-Pitch) Nonlinear System5/Quad System/dot(x1)/1 ==
  X : Inport
  Demux : Demux  Outputs=3
  Selector : Selector  InputPortWidth=4  IndexOptions=Index vector (dialog)  Indices=[1 2 4]  OutputSizes=1
  Subsystem : Subsystem
  x5sin(x1)tan(x2) : Outport
  wires:
  Demux/2 -> Subsystem/2(x2)  "x2"
  X/1 -> Selector/1  "x"
  Demux/1 -> Subsystem/1(x1)  "x1"
  Demux/3 -> Subsystem/3(x5)  "x5"
  Subsystem/1(x5sin(x1)tan(x2)) -> x5sin(x1)tan(x2)/1
  Selector/1 -> Demux/1

== system Quadcopter_nonlinear_Roll_Pitch/Quadcopter 2DOF (Roll-Pitch) Nonlinear System5/Quad System/dot(x1)/Subsystem1 ==
  X : Inport
  Selector : Selector  InputPortWidth=4  IndexOptions=Index vector (dialog)  Indices=[3]  OutputSizes=1
  x4 : Outport
  wires:
  Selector/1 -> x4/1
  X/1 -> Selector/1

== system Quadcopter_nonlinear_Roll_Pitch/Quadcopter 2DOF (Roll-Pitch) Nonlinear System5/Quad System/dot(x2)/1 ==
  X : Inport
  Demux : Demux  Outputs=2
  Selector : Selector  InputPortWidth=4  IndexOptions=Index vector (dialog)  Indices=[1 4]  OutputSizes=1
  Subsystem : Subsystem
  x5cos(x1) : Outport
  wires:
  X/1 -> Selector/1  "x"
  Demux/1 -> Subsystem/1(x1)  "x1"
  Demux/2 -> Subsystem/2(x5)  "x5"
  Subsystem/1(Out1) -> x5cos(x1)/1
  Selector/1 -> Demux/1

== system Quadcopter_nonlinear_Roll_Pitch/Quadcopter 2DOF (Roll-Pitch) Nonlinear System5/Quad System/dot(x4)/1 ==
  X : Inport
  Demux : Demux  Outputs=2
  Selector : Selector  InputPortWidth=4  IndexOptions=Index vector (dialog)  Indices=[1 2]  OutputSizes=1
  Subsystem : Subsystem
  A1cos(x2)sin(x1) : Outport
  wires:
  Demux/1 -> Subsystem/1(x1)  "x1"
  Subsystem/1(A1cos(x2)sin(x1)) -> A1cos(x2)sin(x1)/1
  Demux/2 -> Subsystem/2(x2)  "x2"
  X/1 -> Selector/1  "x"
  Selector/1 -> Demux/1

== system Quadcopter_nonlinear_Roll_Pitch/Quadcopter 2DOF (Roll-Pitch) Nonlinear System5/Quad System/dot(x4)/2 ==
  X : Inport
  Selector : Selector  InputPortWidth=4  IndexOptions=Index vector (dialog)  Indices=[1]  OutputSizes=1
  Subsystem : Subsystem
  Moment a : Outport
  wires:
  Selector/1 -> Subsystem/1(x1)  "x1"
  Subsystem/1(Moment_a) -> Moment a/1
  X/1 -> Selector/1  "x"

== system Quadcopter_nonlinear_Roll_Pitch/Quadcopter 2DOF (Roll-Pitch) Nonlinear System5/Quad System/dot(x4)/3 ==
  X : Inport
  Selector : Selector  InputPortWidth=4  IndexOptions=Index vector (dialog)  Indices=[3]  OutputSizes=1
  Subsystem : Subsystem
  "-A5x4/|x4| " : Outport
  wires:
  Subsystem/1("-A5x4/|x4| ") -> "-A5x4/|x4| "/1
  Selector/1 -> Subsystem/1(x4)
  X/1 -> Selector/1  "x"

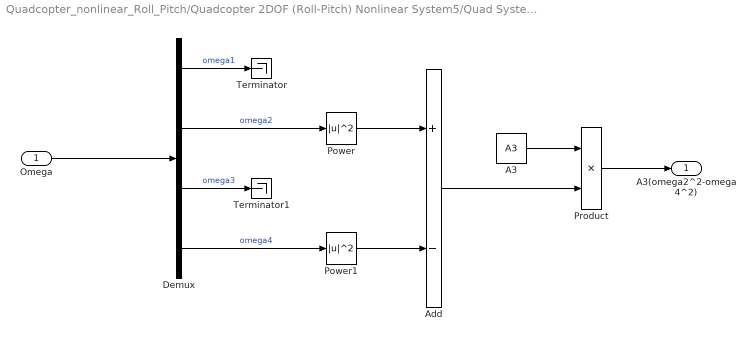
== system Quadcopter_nonlinear_Roll_Pitch/Quadcopter 2DOF (Roll-Pitch) Nonlinear System5/Quad System/dot(x4)/Subsystem ==
  Omega : Inport
  A3 : Constant  Value=A3
  Add : Sum  Inputs=+-
  Demux : Demux
  Power : Math  Operator=magnitude^2  SaturateOnIntegerOverflow=on
  Power1 : Math  Operator=magnitude^2  SaturateOnIntegerOverflow=on
  Product : Product
  Terminator : Terminator
  Terminator1 : Terminator
  A3(omega2^2-omega4^2) : Outport
  wires:
  Product/1 -> A3(omega2^2-omega4^2)/1
  Power1/1 -> Add/2
  Demux/2 -> Power/1  "omega2"
  Demux/4 -> Power1/1  "omega4"
  Add/1 -> Product/2
  Power/1 -> Add/1
  A3/1 -> Product/1
  Omega/1 -> Demux/1
  Demux/3 -> Terminator1/1  "omega3"
  Demux/1 -> Terminator/1  "omega1"

== system Quadcopter_nonlinear_Roll_Pitch/Quadcopter 2DOF (Roll-Pitch) Nonlinear System5/Quad System/dot(x4)/Subsystem1 ==
  X : Inport
  Omega : Inport  Port=2
  A4 : Constant  Value=A4
  Add : Sum  Inputs=+-+-
  Demux : Demux
  Product : Product  Inputs=3
  Selector : Selector  InputPortWidth=4  IndexOptions=Index vector (dialog)  Indices=[4]  OutputSizes=1
  A4x5(omega1-omega2+omega3-omega4) : Outport
  wires:
  Omega/1 -> Demux/1
  Demux/1 -> Add/1  "omega1"
  Demux/2 -> Add/2  "omega2"
  Demux/3 -> Add/3  "omega3"
  Demux/4 -> Add/4  "omega4"
  Add/1 -> Product/1
  A4/1 -> Product/2
  Product/1 -> A4x5(omega1-omega2+omega3-omega4)/1
  Selector/1 -> Product/3
  X/1 -> Selector/1  "x"

== system Quadcopter_nonlinear_Roll_Pitch/Quadcopter 2DOF (Roll-Pitch) Nonlinear System5/Quad System/dot(x5)/1 ==
  X : Inport
  Selector : Selector  InputPortWidth=4  IndexOptions=Index vector (dialog)  Indices=[2]  OutputSizes=1
  Subsystem : Subsystem
  B1sin(x2) : Outport
  wires:
  Subsystem/1(B1sin(x2)) -> B1sin(x2)/1
  Selector/1 -> Subsystem/1(x2)
  X/1 -> Selector/1  "x"

== system Quadcopter_nonlinear_Roll_Pitch/Quadcopter 2DOF (Roll-Pitch) Nonlinear System5/Quad System/dot(x5)/2 ==
  X : Inport
  Selector : Selector  InputPortWidth=4  IndexOptions=Index vector (dialog)  Indices=[2]  OutputSizes=1
  Subsystem : Subsystem
  Moment_a : Outport
  wires:
  X/1 -> Selector/1  "x"
  Subsystem/1(moment_a) -> Moment_a/1
  Selector/1 -> Subsystem/1(In1)

== system Quadcopter_nonlinear_Roll_Pitch/Quadcopter 2DOF (Roll-Pitch) Nonlinear System5/Quad System/dot(x5)/3 ==
  X : Inport
  Selector : Selector  InputPortWidth=4  IndexOptions=Index vector (dialog)  Indices=[4]  OutputSizes=1
  Subsystem : Subsystem
  "-B5x5/|x5| " : Outport
  wires:
  Selector/1 -> Subsystem/1(x5)  "x5"
  Subsystem/1("-B5x5/|x5| ") -> "-B5x5/|x5| "/1
  X/1 -> Selector/1  "x"

== system Quadcopter_nonlinear_Roll_Pitch/Quadcopter 2DOF (Roll-Pitch) Nonlinear System5/Quad System/dot(x5)/Subsystem ==
  Omega : Inport
  Add : Sum  Inputs=+-
  B3 : Constant  Value=(b * d_cg) / (m_tot * h_cg^2 + J_yy)
  Demux : Demux
  Power : Math  Operator=magnitude^2  SaturateOnIntegerOverflow=on
  Power1 : Math  Operator=magnitude^2  SaturateOnIntegerOverflow=on
  Product : Product
  Terminator : Terminator
  Terminator1 : Terminator
  B3(omega1^2-omega3^2) : Outport
  wires:
  Product/1 -> B3(omega1^2-omega3^2)/1
  Power1/1 -> Add/2
  Add/1 -> Product/2
  Power/1 -> Add/1
  B3/1 -> Product/1
  Omega/1 -> Demux/1
  Demux/3 -> Power1/1  "omega3"
  Demux/1 -> Power/1  "omega1"
  Demux/2 -> Terminator/1  "omega2"
  Demux/4 -> Terminator1/1  "omega4"

== system Quadcopter_nonlinear_Roll_Pitch/Quadcopter 2DOF (Roll-Pitch) Nonlinear System5/Quad System/dot(x5)/Subsystem1 ==
  X : Inport
  Omega : Inport  Port=2
  Add : Sum  Inputs=+-+-
  B4 : Constant  Value=(-J_R) / (m_tot * h_cg^2 + J_yy)
  Demux : Demux
  Product : Product  Inputs=3
  Selector : Selector  InputPortWidth=4  IndexOptions=Index vector (dialog)  Indices=[3]  OutputSizes=1
  B4x4(omega1-omega2+omega3-omega4) : Outport
  wires:
  Omega/1 -> Demux/1
  Demux/1 -> Add/1  "omega1"
  Demux/2 -> Add/2  "omega2"
  Demux/3 -> Add/3  "omega3"
  Demux/4 -> Add/4  "omega4"
  Add/1 -> Product/1
  B4/1 -> Product/2
  Product/1 -> B4x4(omega1-omega2+omega3-omega4)/1
  Selector/1 -> Product/3
  X/1 -> Selector/1  "x"

== system Quadcopter_nonlinear_Roll_Pitch/Quadcopter 2DOF (Roll-Pitch) Nonlinear System6/Quad System/dot(x1)/1 ==
  X : Inport
  Demux : Demux  Outputs=3
  Selector : Selector  InputPortWidth=4  IndexOptions=Index vector (dialog)  Indices=[1 2 4]  OutputSizes=1
  Subsystem : Subsystem
  x5sin(x1)tan(x2) : Outport
  wires:
  Demux/2 -> Subsystem/2(x2)  "x2"
  X/1 -> Selector/1  "x"
  Demux/1 -> Subsystem/1(x1)  "x1"
  Demux/3 -> Subsystem/3(x5)  "x5"
  Subsystem/1(x5sin(x1)tan(x2)) -> x5sin(x1)tan(x2)/1
  Selector/1 -> Demux/1

== system Quadcopter_nonlinear_Roll_Pitch/Quadcopter 2DOF (Roll-Pitch) Nonlinear System6/Quad System/dot(x1)/Subsystem1 ==
  X : Inport
  Selector : Selector  InputPortWidth=4  IndexOptions=Index vector (dialog)  Indices=[3]  OutputSizes=1
  x4 : Outport
  wires:
  Selector/1 -> x4/1
  X/1 -> Selector/1

== system Quadcopter_nonlinear_Roll_Pitch/Quadcopter 2DOF (Roll-Pitch) Nonlinear System6/Quad System/dot(x2)/1 ==
  X : Inport
  Demux : Demux  Outputs=2
  Selector : Selector  InputPortWidth=4  IndexOptions=Index vector (dialog)  Indices=[1 4]  OutputSizes=1
  Subsystem : Subsystem
  x5cos(x1) : Outport
  wires:
  X/1 -> Selector/1  "x"
  Demux/1 -> Subsystem/1(x1)  "x1"
  Demux/2 -> Subsystem/2(x5)  "x5"
  Subsystem/1(Out1) -> x5cos(x1)/1
  Selector/1 -> Demux/1

== system Quadcopter_nonlinear_Roll_Pitch/Quadcopter 2DOF (Roll-Pitch) Nonlinear System6/Quad System/dot(x4)/1 ==
  X : Inport
  Demux : Demux  Outputs=2
  Selector : Selector  InputPortWidth=4  IndexOptions=Index vector (dialog)  Indices=[1 2]  OutputSizes=1
  Subsystem : Subsystem
  A1cos(x2)sin(x1) : Outport
  wires:
  Demux/1 -> Subsystem/1(x1)  "x1"
  Subsystem/1(A1cos(x2)sin(x1)) -> A1cos(x2)sin(x1)/1
  Demux/2 -> Subsystem/2(x2)  "x2"
  X/1 -> Selector/1  "x"
  Selector/1 -> Demux/1

== system Quadcopter_nonlinear_Roll_Pitch/Quadcopter 2DOF (Roll-Pitch) Nonlinear System6/Quad System/dot(x4)/2 ==
  X : Inport
  Selector : Selector  InputPortWidth=4  IndexOptions=Index vector (dialog)  Indices=[1]  OutputSizes=1
  Subsystem : Subsystem
  Moment a : Outport
  wires:
  Selector/1 -> Subsystem/1(x1)  "x1"
  Subsystem/1(Moment_a) -> Moment a/1
  X/1 -> Selector/1  "x"

== system Quadcopter_nonlinear_Roll_Pitch/Quadcopter 2DOF (Roll-Pitch) Nonlinear System6/Quad System/dot(x4)/3 ==
  X : Inport
  Selector : Selector  InputPortWidth=4  IndexOptions=Index vector (dialog)  Indices=[3]  OutputSizes=1
  Subsystem : Subsystem
  "-A5x4/|x4| " : Outport
  wires:
  Subsystem/1("-A5x4/|x4| ") -> "-A5x4/|x4| "/1
  Selector/1 -> Subsystem/1(x4)
  X/1 -> Selector/1  "x"

== system Quadcopter_nonlinear_Roll_Pitch/Quadcopter 2DOF (Roll-Pitch) Nonlinear System6/Quad System/dot(x4)/Subsystem ==
  Omega : Inport
  A3 : Constant  Value=A3
  Add : Sum  Inputs=+-
  Demux : Demux
  Power : Math  Operator=magnitude^2  SaturateOnIntegerOverflow=on
  Power1 : Math  Operator=magnitude^2  SaturateOnIntegerOverflow=on
  Product : Product
  Terminator : Terminator
  Terminator1 : Terminator
  A3(omega2^2-omega4^2) : Outport
  wires:
  Product/1 -> A3(omega2^2-omega4^2)/1
  Power1/1 -> Add/2
  Demux/2 -> Power/1  "omega2"
  Demux/4 -> Power1/1  "omega4"
  Add/1 -> Product/2
  Power/1 -> Add/1
  A3/1 -> Product/1
  Omega/1 -> Demux/1
  Demux/3 -> Terminator1/1  "omega3"
  Demux/1 -> Terminator/1  "omega1"

== system Quadcopter_nonlinear_Roll_Pitch/Quadcopter 2DOF (Roll-Pitch) Nonlinear System6/Quad System/dot(x4)/Subsystem1 ==
  X : Inport
  Omega : Inport  Port=2
  A4 : Constant  Value=A4
  Add : Sum  Inputs=+-+-
  Demux : Demux
  Product : Product  Inputs=3
  Selector : Selector  InputPortWidth=4  IndexOptions=Index vector (dialog)  Indices=[4]  OutputSizes=1
  A4x5(omega1-omega2+omega3-omega4) : Outport
  wires:
  Omega/1 -> Demux/1
  Demux/1 -> Add/1  "omega1"
  Demux/2 -> Add/2  "omega2"
  Demux/3 -> Add/3  "omega3"
  Demux/4 -> Add/4  "omega4"
  Add/1 -> Product/1
  A4/1 -> Product/2
  Product/1 -> A4x5(omega1-omega2+omega3-omega4)/1
  Selector/1 -> Product/3
  X/1 -> Selector/1  "x"

== system Quadcopter_nonlinear_Roll_Pitch/Quadcopter 2DOF (Roll-Pitch) Nonlinear System6/Quad System/dot(x5)/1 ==
  X : Inport
  Selector : Selector  InputPortWidth=4  IndexOptions=Index vector (dialog)  Indices=[2]  OutputSizes=1
  Subsystem : Subsystem
  B1sin(x2) : Outport
  wires:
  Subsystem/1(B1sin(x2)) -> B1sin(x2)/1
  Selector/1 -> Subsystem/1(x2)
  X/1 -> Selector/1  "x"

== system Quadcopter_nonlinear_Roll_Pitch/Quadcopter 2DOF (Roll-Pitch) Nonlinear System6/Quad System/dot(x5)/2 ==
  X : Inport
  Selector : Selector  InputPortWidth=4  IndexOptions=Index vector (dialog)  Indices=[2]  OutputSizes=1
  Subsystem : Subsystem
  Moment_a : Outport
  wires:
  X/1 -> Selector/1  "x"
  Subsystem/1(moment_a) -> Moment_a/1
  Selector/1 -> Subsystem/1(In1)

== system Quadcopter_nonlinear_Roll_Pitch/Quadcopter 2DOF (Roll-Pitch) Nonlinear System6/Quad System/dot(x5)/3 ==
  X : Inport
  Selector : Selector  InputPortWidth=4  IndexOptions=Index vector (dialog)  Indices=[4]  OutputSizes=1
  Subsystem : Subsystem
  "-B5x5/|x5| " : Outport
  wires:
  Selector/1 -> Subsystem/1(x5)  "x5"
  Subsystem/1("-B5x5/|x5| ") -> "-B5x5/|x5| "/1
  X/1 -> Selector/1  "x"

== system Quadcopter_nonlinear_Roll_Pitch/Quadcopter 2DOF (Roll-Pitch) Nonlinear System6/Quad System/dot(x5)/Subsystem ==
  Omega : Inport
  Add : Sum  Inputs=+-
  B3 : Constant  Value=(b * d_cg) / (m_tot * h_cg^2 + J_yy)
  Demux : Demux
  Power : Math  Operator=magnitude^2  SaturateOnIntegerOverflow=on
  Power1 : Math  Operator=magnitude^2  SaturateOnIntegerOverflow=on
  Product : Product
  Terminator : Terminator
  Terminator1 : Terminator
  B3(omega1^2-omega3^2) : Outport
  wires:
  Product/1 -> B3(omega1^2-omega3^2)/1
  Power1/1 -> Add/2
  Add/1 -> Product/2
  Power/1 -> Add/1
  B3/1 -> Product/1
  Omega/1 -> Demux/1
  Demux/3 -> Power1/1  "omega3"
  Demux/1 -> Power/1  "omega1"
  Demux/2 -> Terminator/1  "omega2"
  Demux/4 -> Terminator1/1  "omega4"

== system Quadcopter_nonlinear_Roll_Pitch/Quadcopter 2DOF (Roll-Pitch) Nonlinear System6/Quad System/dot(x5)/Subsystem1 ==
  X : Inport
  Omega : Inport  Port=2
  Add : Sum  Inputs=+-+-
  B4 : Constant  Value=(-J_R) / (m_tot * h_cg^2 + J_yy)
  Demux : Demux
  Product : Product  Inputs=3
  Selector : Selector  InputPortWidth=4  IndexOptions=Index vector (dialog)  Indices=[3]  OutputSizes=1
  B4x4(omega1-omega2+omega3-omega4) : Outport
  wires:
  Omega/1 -> Demux/1
  Demux/1 -> Add/1  "omega1"
  Demux/2 -> Add/2  "omega2"
  Demux/3 -> Add/3  "omega3"
  Demux/4 -> Add/4  "omega4"
  Add/1 -> Product/1
  B4/1 -> Product/2
  Product/1 -> B4x4(omega1-omega2+omega3-omega4)/1
  Selector/1 -> Product/3
  X/1 -> Selector/1  "x"

== system Quadcopter_nonlinear_Roll_Pitch/Quadcopter 2DOF (Roll-Pitch) Nonlinear System7/Quad System/dot(x1)/1 ==
  X : Inport
  Demux : Demux  Outputs=3
  Selector : Selector  InputPortWidth=4  IndexOptions=Index vector (dialog)  Indices=[1 2 4]  OutputSizes=1
  Subsystem : Subsystem
  x5sin(x1)tan(x2) : Outport
  wires:
  Demux/2 -> Subsystem/2(x2)  "x2"
  X/1 -> Selector/1  "x"
  Demux/1 -> Subsystem/1(x1)  "x1"
  Demux/3 -> Subsystem/3(x5)  "x5"
  Subsystem/1(x5sin(x1)tan(x2)) -> x5sin(x1)tan(x2)/1
  Selector/1 -> Demux/1

== system Quadcopter_nonlinear_Roll_Pitch/Quadcopter 2DOF (Roll-Pitch) Nonlinear System7/Quad System/dot(x1)/Subsystem1 ==
  X : Inport
  Selector : Selector  InputPortWidth=4  IndexOptions=Index vector (dialog)  Indices=[3]  OutputSizes=1
  x4 : Outport
  wires:
  Selector/1 -> x4/1
  X/1 -> Selector/1

== system Quadcopter_nonlinear_Roll_Pitch/Quadcopter 2DOF (Roll-Pitch) Nonlinear System7/Quad System/dot(x2)/1 ==
  X : Inport
  Demux : Demux  Outputs=2
  Selector : Selector  InputPortWidth=4  IndexOptions=Index vector (dialog)  Indices=[1 4]  OutputSizes=1
  Subsystem : Subsystem
  x5cos(x1) : Outport
  wires:
  X/1 -> Selector/1  "x"
  Demux/1 -> Subsystem/1(x1)  "x1"
  Demux/2 -> Subsystem/2(x5)  "x5"
  Subsystem/1(Out1) -> x5cos(x1)/1
  Selector/1 -> Demux/1

== system Quadcopter_nonlinear_Roll_Pitch/Quadcopter 2DOF (Roll-Pitch) Nonlinear System7/Quad System/dot(x4)/1 ==
  X : Inport
  Demux : Demux  Outputs=2
  Selector : Selector  InputPortWidth=4  IndexOptions=Index vector (dialog)  Indices=[1 2]  OutputSizes=1
  Subsystem : Subsystem
  A1cos(x2)sin(x1) : Outport
  wires:
  Demux/1 -> Subsystem/1(x1)  "x1"
  Subsystem/1(A1cos(x2)sin(x1)) -> A1cos(x2)sin(x1)/1
  Demux/2 -> Subsystem/2(x2)  "x2"
  X/1 -> Selector/1  "x"
  Selector/1 -> Demux/1

== system Quadcopter_nonlinear_Roll_Pitch/Quadcopter 2DOF (Roll-Pitch) Nonlinear System7/Quad System/dot(x4)/2 ==
  X : Inport
  Selector : Selector  InputPortWidth=4  IndexOptions=Index vector (dialog)  Indices=[1]  OutputSizes=1
  Subsystem : Subsystem
  Moment a : Outport
  wires:
  Selector/1 -> Subsystem/1(x1)  "x1"
  Subsystem/1(Moment_a) -> Moment a/1
  X/1 -> Selector/1  "x"

== system Quadcopter_nonlinear_Roll_Pitch/Quadcopter 2DOF (Roll-Pitch) Nonlinear System7/Quad System/dot(x4)/3 ==
  X : Inport
  Selector : Selector  InputPortWidth=4  IndexOptions=Index vector (dialog)  Indices=[3]  OutputSizes=1
  Subsystem : Subsystem
  "-A5x4/|x4| " : Outport
  wires:
  Subsystem/1("-A5x4/|x4| ") -> "-A5x4/|x4| "/1
  Selector/1 -> Subsystem/1(x4)
  X/1 -> Selector/1  "x"

== system Quadcopter_nonlinear_Roll_Pitch/Quadcopter 2DOF (Roll-Pitch) Nonlinear System7/Quad System/dot(x4)/Subsystem ==
  Omega : Inport
  A3 : Constant  Value=A3
  Add : Sum  Inputs=+-
  Demux : Demux
  Power : Math  Operator=magnitude^2  SaturateOnIntegerOverflow=on
  Power1 : Math  Operator=magnitude^2  SaturateOnIntegerOverflow=on
  Product : Product
  Terminator : Terminator
  Terminator1 : Terminator
  A3(omega2^2-omega4^2) : Outport
  wires:
  Product/1 -> A3(omega2^2-omega4^2)/1
  Power1/1 -> Add/2
  Demux/2 -> Power/1  "omega2"
  Demux/4 -> Power1/1  "omega4"
  Add/1 -> Product/2
  Power/1 -> Add/1
  A3/1 -> Product/1
  Omega/1 -> Demux/1
  Demux/3 -> Terminator1/1  "omega3"
  Demux/1 -> Terminator/1  "omega1"

== system Quadcopter_nonlinear_Roll_Pitch/Quadcopter 2DOF (Roll-Pitch) Nonlinear System7/Quad System/dot(x4)/Subsystem1 ==
  X : Inport
  Omega : Inport  Port=2
  A4 : Constant  Value=A4
  Add : Sum  Inputs=+-+-
  Demux : Demux
  Product : Product  Inputs=3
  Selector : Selector  InputPortWidth=4  IndexOptions=Index vector (dialog)  Indices=[4]  OutputSizes=1
  A4x5(omega1-omega2+omega3-omega4) : Outport
  wires:
  Omega/1 -> Demux/1
  Demux/1 -> Add/1  "omega1"
  Demux/2 -> Add/2  "omega2"
  Demux/3 -> Add/3  "omega3"
  Demux/4 -> Add/4  "omega4"
  Add/1 -> Product/1
  A4/1 -> Product/2
  Product/1 -> A4x5(omega1-omega2+omega3-omega4)/1
  Selector/1 -> Product/3
  X/1 -> Selector/1  "x"

== system Quadcopter_nonlinear_Roll_Pitch/Quadcopter 2DOF (Roll-Pitch) Nonlinear System7/Quad System/dot(x5)/1 ==
  X : Inport
  Selector : Selector  InputPortWidth=4  IndexOptions=Index vector (dialog)  Indices=[2]  OutputSizes=1
  Subsystem : Subsystem
  B1sin(x2) : Outport
  wires:
  Subsystem/1(B1sin(x2)) -> B1sin(x2)/1
  Selector/1 -> Subsystem/1(x2)
  X/1 -> Selector/1  "x"

== system Quadcopter_nonlinear_Roll_Pitch/Quadcopter 2DOF (Roll-Pitch) Nonlinear System7/Quad System/dot(x5)/2 ==
  X : Inport
  Selector : Selector  InputPortWidth=4  IndexOptions=Index vector (dialog)  Indices=[2]  OutputSizes=1
  Subsystem : Subsystem
  Moment_a : Outport
  wires:
  X/1 -> Selector/1  "x"
  Subsystem/1(moment_a) -> Moment_a/1
  Selector/1 -> Subsystem/1(In1)

== system Quadcopter_nonlinear_Roll_Pitch/Quadcopter 2DOF (Roll-Pitch) Nonlinear System7/Quad System/dot(x5)/3 ==
  X : Inport
  Selector : Selector  InputPortWidth=4  IndexOptions=Index vector (dialog)  Indices=[4]  OutputSizes=1
  Subsystem : Subsystem
  "-B5x5/|x5| " : Outport
  wires:
  Selector/1 -> Subsystem/1(x5)  "x5"
  Subsystem/1("-B5x5/|x5| ") -> "-B5x5/|x5| "/1
  X/1 -> Selector/1  "x"

== system Quadcopter_nonlinear_Roll_Pitch/Quadcopter 2DOF (Roll-Pitch) Nonlinear System7/Quad System/dot(x5)/Subsystem ==
  Omega : Inport
  Add : Sum  Inputs=+-
  B3 : Constant  Value=(b * d_cg) / (m_tot * h_cg^2 + J_yy)
  Demux : Demux
  Power : Math  Operator=magnitude^2  SaturateOnIntegerOverflow=on
  Power1 : Math  Operator=magnitude^2  SaturateOnIntegerOverflow=on
  Product : Product
  Terminator : Terminator
  Terminator1 : Terminator
  B3(omega1^2-omega3^2) : Outport
  wires:
  Product/1 -> B3(omega1^2-omega3^2)/1
  Power1/1 -> Add/2
  Add/1 -> Product/2
  Power/1 -> Add/1
  B3/1 -> Product/1
  Omega/1 -> Demux/1
  Demux/3 -> Power1/1  "omega3"
  Demux/1 -> Power/1  "omega1"
  Demux/2 -> Terminator/1  "omega2"
  Demux/4 -> Terminator1/1  "omega4"

== system Quadcopter_nonlinear_Roll_Pitch/Quadcopter 2DOF (Roll-Pitch) Nonlinear System7/Quad System/dot(x5)/Subsystem1 ==
  X : Inport
  Omega : Inport  Port=2
  Add : Sum  Inputs=+-+-
  B4 : Constant  Value=(-J_R) / (m_tot * h_cg^2 + J_yy)
  Demux : Demux
  Product : Product  Inputs=3
  Selector : Selector  InputPortWidth=4  IndexOptions=Index vector (dialog)  Indices=[3]  OutputSizes=1
  B4x4(omega1-omega2+omega3-omega4) : Outport
  wires:
  Omega/1 -> Demux/1
  Demux/1 -> Add/1  "omega1"
  Demux/2 -> Add/2  "omega2"
  Demux/3 -> Add/3  "omega3"
  Demux/4 -> Add/4  "omega4"
  Add/1 -> Product/1
  B4/1 -> Product/2
  Product/1 -> B4x4(omega1-omega2+omega3-omega4)/1
  Selector/1 -> Product/3
  X/1 -> Selector/1  "x"

== system Quadcopter_nonlinear_Roll_Pitch/Quadcopter 2DOF (Roll-Pitch) Nonlinear System8/Quad System/dot(x1)/1 ==
  X : Inport
  Demux : Demux  Outputs=3
  Selector : Selector  InputPortWidth=4  IndexOptions=Index vector (dialog)  Indices=[1 2 4]  OutputSizes=1
  Subsystem : Subsystem
  x5sin(x1)tan(x2) : Outport
  wires:
  Demux/2 -> Subsystem/2(x2)  "x2"
  X/1 -> Selector/1  "x"
  Demux/1 -> Subsystem/1(x1)  "x1"
  Demux/3 -> Subsystem/3(x5)  "x5"
  Subsystem/1(x5sin(x1)tan(x2)) -> x5sin(x1)tan(x2)/1
  Selector/1 -> Demux/1
